simulink model "initial_test"  (R2019b)
settings: Solver=FixedStepAuto  StartTime=0.0  StopTime=Inf  FixedStep=FIXED_STEP_SIZE  RelTol=1e-3
values from neighbouring files (symbols this model uses):
  GAZEBO_SYNC_DT = 0.01    [initial_test_script.m]
undefined symbols (not defined in the file or in its folder): Angular, Linear
libraries: robotlib x4, simulink x3, robotgazebolib x1
settings Model: SimulationMode=external  Creator=ananda  LastModifiedBy=ananda
settings OptimizationCC: EnhancedBackFolding=on  PassReuseOutputArgsAs=Individual arguments  ZeroExternalMemoryAtStartup=off  ZeroInternalMemoryAtStartup=off  MaxStackSize=64  OptimizeBlockOrder=speed  DifferentSizesBufferReuse=on  OptimizationCustomize=off  EfficientTunableParamExpr=on
settings DebuggingCC: ParameterTunabilityLossMsg=error
settings HardwareCC: ProdBitPerPointer=32  ProdBitPerSizeT=32  ProdBitPerPtrDiffT=32  ProdLargestAtomicFloat=None  ProdIntDivRoundTo=Undefined  ProdEndianess=Unspecified  ProdWordSize=32  ProdHWDeviceType=Generic->Unspecified (assume 32-bit Generic)  UseEmbeddedCoderFeatures=off
settings SFSimCC: MATLABDynamicMemAlloc=off
settings RTWCC: SystemTargetFile=ert.tlc  HardwareBoard=Robot Operating System (ROS)  TLCOptions="-aInlineSetEventsForThisBaseRateFcn=TLC_FALSE -aSuppressMultiTaskScheduler=TLC_FALSE  -aRateBasedStepFcn=0"  TemplateMakefile=ert_default_tmf  GenerateReport=on  Toolchain=Catkin  IncludeHyperlinkInReport=on  LaunchReport=on  TargetLang=C++  GenerateTraceInfo=on  GenerateTraceReport=on  GenerateTraceReportSl=on  GenerateTraceReportSf=on  GenerateTraceReportEml=on
settings CodeAppCC: ForceParamTrailComments=on  IgnoreCustomStorageClasses=off  OperatorAnnotations=on  SimulinkDataObjDesc=on  SFDataObjDesc=on  InsertBlockDesc=on
settings ERTTargetCC: SupportNonInlinedSFcns=on

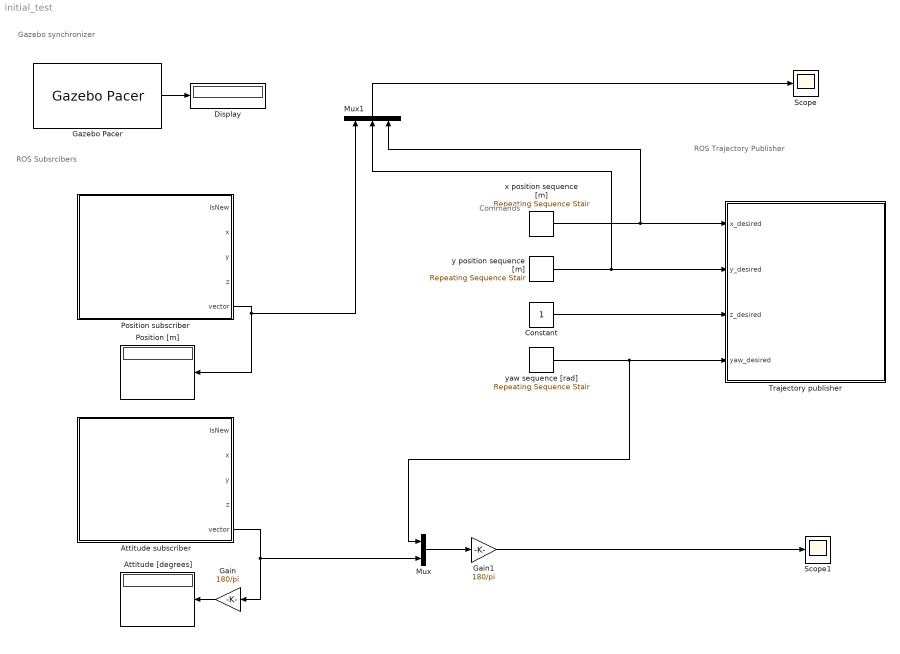
== system initial_test ==
  note: Commands
  note: ROS Trajectory Publisher
  note: Gazebo synchronizer
  note: ROS Subsrcibers
  Attitude [degrees] : Display
  Attitude subscriber : Subsystem
  Constant : Constant
  Display : Display
  Gain : Gain  Gain=180/pi
  Gain1 : Gain  Gain=180/pi
  Gazebo Pacer : robotgazebolib/Gazebo Pacer  ResetBehavior=Reset Gazebo simulation time  SampleTime=GAZEBO_SYNC_DT
      settings: SourceProductName=Robotics System Toolbox  SourceProductBaseCode=RO
  Mux : Mux  Inputs=2
  Mux1 : Mux  Inputs=3
  Position [m] : Display
  Position subscriber : Subsystem
  Scope : Scope
  Scope1 : Scope
  Trajectory publisher : Subsystem
  x position sequence [m] : simulink/Sources/Repeating Sequence Stair  OutValues=[0 1 1 1 1 1 0 0 0].'  tsamp=3  OutMin=[]  OutMax=[]  OutDataTypeStr=double  OutputDataTypeScalingMode=double  OutDataType=fixdt(0,8)  ConRadixGroup=Best Precision: Vector-wise  OutScaling=2^-12
  y position sequence [m] : simulink/Sources/Repeating Sequence Stair  OutValues=[0 0 1 1 1 1 1 0 0].'  tsamp=3  OutMin=[]  OutMax=[]  OutDataTypeStr=double  OutputDataTypeScalingMode=double  OutDataType=fixdt(0,8)  ConRadixGroup=Best Precision: Vector-wise  OutScaling=2^-12
  yaw sequence [rad] : simulink/Sources/Repeating Sequence Stair  OutValues=[0 0 0 1 -1 0 0 0 0 0].'  tsamp=3  OutMin=[]  OutMax=[]  OutDataTypeStr=double  OutputDataTypeScalingMode=double  OutDataType=fixdt(0,8)  ConRadixGroup=Best Precision: Vector-wise  OutScaling=2^-12
  wires:
  x position sequence [m]/1 -> Trajectory publisher/1(x_desired), Mux1/3
  y position sequence [m]/1 -> Trajectory publisher/2(y_desired), Mux1/2
  Position subscriber/5(vector) -> Mux1/1, Position [m]/1
  Constant/1 -> Trajectory publisher/3(z_desired)
  yaw sequence [rad]/1 -> Mux/1, Trajectory publisher/4(yaw_desired)
  Attitude subscriber/5(vector) -> Gain/1, Mux/2
  Gain/1 -> Attitude [degrees]/1
  Mux/1 -> Gain1/1
  Gain1/1 -> Scope1/1
  Gazebo Pacer/1 -> Display/1
  Mux1/1 -> Scope/1

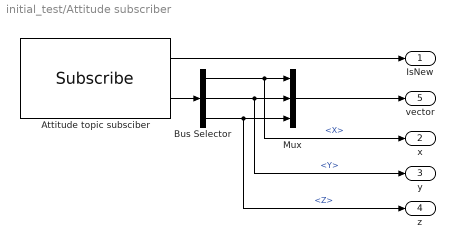
== system initial_test/Attitude subscriber ==
  Attitude topic subsciber : robotlib/Subscribe  topicSource=Specify your own  topic=/hummingbird/orientation_rpy  messageType=geometry_msgs/Vector3  sampleTime=ATTI_SUB_DT  messageQueueLength=1
      settings: SourceProductName=ROS Toolbox
  Bus Selector : BusSelector  OutputSignals=X,Y,Z
  Mux : Mux  Inputs=3
  IsNew : Outport
  x : Outport  Port=2
  y : Outport  Port=3
  z : Outport  Port=4
  vector : Outport  Port=5
  wires:
  Bus Selector/3 -> z/1, Mux/3  "<Z>"
  Bus Selector/2 -> y/1, Mux/2  "<Y>"
  Bus Selector/1 -> x/1, Mux/1  "<X>"
  Attitude topic subsciber/2 -> Bus Selector/1
  Attitude topic subsciber/1 -> IsNew/1
  Mux/1 -> vector/1

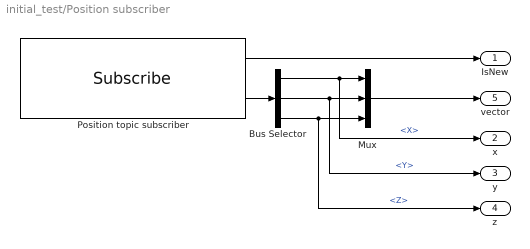
== system initial_test/Position subscriber ==
  Bus Selector : BusSelector  OutputSignals=Point.X,Point.Y,Point.Z
  Mux : Mux  Inputs=3
  Position topic subscriber : robotlib/Subscribe  topicSource=Specify your own  topic=/hummingbird/odometry_sensor1/position  messageType=geometry_msgs/PointStamped  sampleTime=POS_SUB_DT  messageQueueLength=1
      settings: SourceProductName=ROS Toolbox
  IsNew : Outport
  x : Outport  Port=2
  y : Outport  Port=3
  z : Outport  Port=4
  vector : Outport  Port=5
  wires:
  Bus Selector/3 -> z/1, Mux/3  "<Z>"
  Bus Selector/2 -> y/1, Mux/2  "<Y>"
  Mux/1 -> vector/1
  Bus Selector/1 -> x/1, Mux/1  "<X>"
  Position topic subscriber/2 -> Bus Selector/1
  Position topic subscriber/1 -> IsNew/1

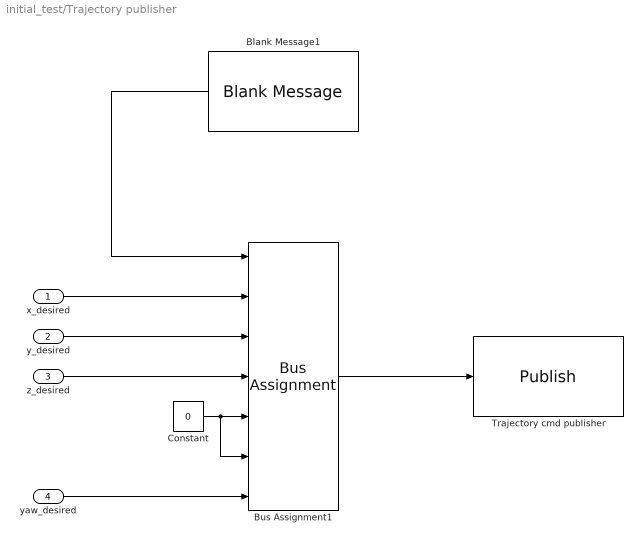
== system initial_test/Trajectory publisher ==
  x_desired : Inport
  y_desired : Inport  Port=2
  z_desired : Inport  Port=3
  yaw_desired : Inport  Port=4
  Blank Message1 : robotlib/Blank Message  messageClass=Message  entityType=geometry_msgs/Twist  messageType=geometry_msgs/Twist  SampleTime=inf
      settings: SourceProductName=ROS Toolbox
  Bus Assignment1 : BusAssignment  AssignedSignals=Linear.X,Linear.Y,Linear.Z,Angular.X,Angular.Y,Angular.Z
  Constant : Constant  Value=0
  Trajectory cmd publisher : robotlib/Publish  topicSource=Specify your own  topic=/matlab/tracejtoryTwist  messageType=geometry_msgs/Twist  messageQueueLength=1
      settings: SourceProductName=ROS Toolbox
  wires:
  Blank Message1/1 -> Bus Assignment1/1
  Constant/1 -> Bus Assignment1/6, Bus Assignment1/5
  Bus Assignment1/1 -> Trajectory cmd publisher/1
  x_desired/1 -> Bus Assignment1/2
  y_desired/1 -> Bus Assignment1/3
  z_desired/1 -> Bus Assignment1/4
  yaw_desired/1 -> Bus Assignment1/7
